simulink subsystem "JerkMetrics"  (R2023b)
settings: Solver=VariableStepAuto  StartTime=0.0  StopTime=10.0  RelTol=1e-3
undefined symbols (not defined in the file): assessment
settings Model: Creator=The MathWorks, Inc.  LastModifiedBy=The MathWorks, Inc.
settings SolverCC: MaxZcPerStep=1
settings DebuggingCC: UnconnectedInputMsg=warning  UnconnectedOutputMsg=warning  UnconnectedLineMsg=warning  SubsystemReferenceDiagnosticForUnitTest=warning
settings ModelReferenceCC: EnableRefExpFcnMdlSchedulingChecks=on
settings RTWCC: DLArmComputeVersion=19.05

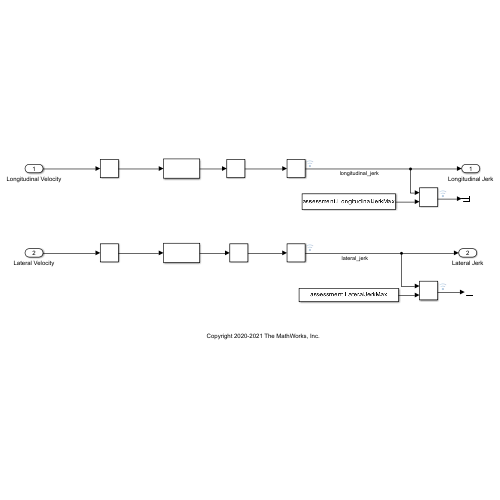
[thumbnail: Simulink's stored preview of the top-level diagram]
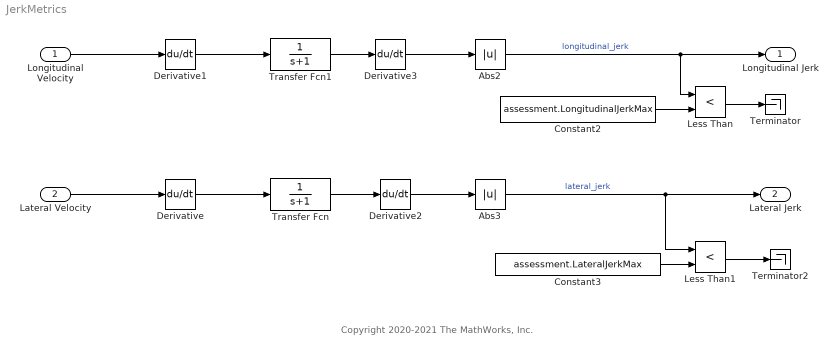
== system JerkMetrics ==
  note: Copyright 2020-2021 The MathWorks, Inc.
  Longitudinal Velocity : Inport
  Lateral Velocity : Inport  Port=2
  Abs2 : Abs  ZeroCross=off  SaturateOnIntegerOverflow=off
  Abs3 : Abs  ZeroCross=off  SaturateOnIntegerOverflow=off
  Constant2 : Constant  Value=assessment.LongitudinalJerkMax
  Constant3 : Constant  Value=assessment.LateralJerkMax
  Derivative : Derivative  CoefficientInTFapproximation=1
  Derivative1 : Derivative  CoefficientInTFapproximation=10
  Derivative2 : Derivative  CoefficientInTFapproximation=1
  Derivative3 : Derivative  CoefficientInTFapproximation=10
  Less Than : RelationalOperator  Operator=<  OutDataTypeStr=boolean  RndMeth=Simplest  InputSameDT=off
  Less Than1 : RelationalOperator  Operator=<  OutDataTypeStr=boolean  RndMeth=Simplest  InputSameDT=off
  Terminator : Terminator
  Terminator2 : Terminator
  Transfer Fcn : TransferFcn  Denominator=[1 1]
  Transfer Fcn1 : TransferFcn  Denominator=[1 1]
  Longitudinal Jerk : Outport
  Lateral Jerk : Outport  Port=2
  wires:
  Abs3/1 -> Less Than1/1, Lateral Jerk/1  "lateral_jerk"
  Derivative1/1 -> Transfer Fcn1/1
  Transfer Fcn1/1 -> Derivative3/1
  Derivative/1 -> Transfer Fcn/1
  Abs2/1 -> Less Than/1, Longitudinal Jerk/1  "longitudinal_jerk"
  Derivative3/1 -> Abs2/1
  Less Than1/1 -> Terminator2/1
  Derivative2/1 -> Abs3/1
  Transfer Fcn/1 -> Derivative2/1
  Constant2/1 -> Less Than/2
  Less Than/1 -> Terminator/1
  Constant3/1 -> Less Than1/2
  Longitudinal Velocity/1 -> Derivative1/1
  Lateral Velocity/1 -> Derivative/1
